simulink model "block_model"  (R2020a)
settings: Solver=VariableStepAuto  StartTime=0.0  StopTime=30  RelTol=1e-3
undefined symbols (not defined in the file or in its folder): DiscIntNeverNeededParam
libraries: simulink x6
settings Model: Creator=igorbeduin  LastModifiedBy=igorbeduin
settings SFSimCC: CustomCodeUndefinedFunction=UseInterfaceOnly

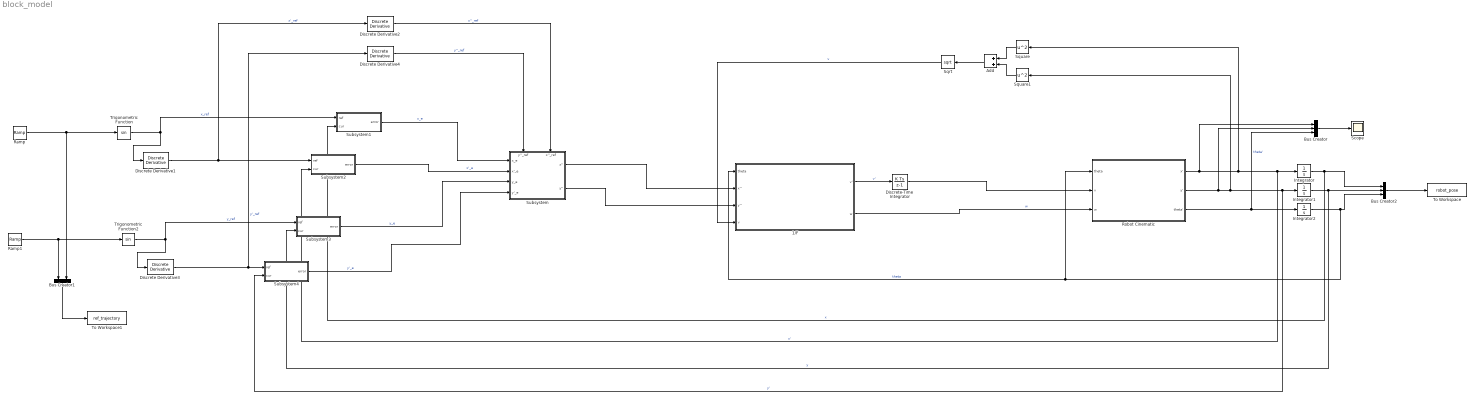
== system block_model ==
  1/F : Subsystem
  Add : Sum
  Bus Creator : BusCreator  Inputs=3
  Bus Creator1 : BusCreator  Inputs=2
  Bus Creator2 : BusCreator  Inputs=3
  Discrete Derivative{1..4} (4 alike) : simulink/Discrete/Discrete Derivative  gainval=1.0  ICPrevScaledInput=0.0  OutMin=[]  OutMax=[]  OutDataType=fixdt(1, 16)  OutScaling=2^-10  DoSatur=off
  Discrete-Time Integrator : DiscreteIntegrator  SampleTime=-1  ICPrevOutput=DiscIntNeverNeededParam  ICPrevScaledInput=DiscIntNeverNeededParam
  Integrator : Integrator
  Integrator1 : Integrator
  Integrator2 : Integrator
  Ramp : simulink/Sources/Ramp  slope=1  start=0  InitialOutput=0
  Ramp1 : simulink/Sources/Ramp  slope=2  start=0  InitialOutput=0
  Robot Cinematic : Subsystem
  Scope : Scope
  Sqrt : Sqrt  SaturateOnIntegerOverflow=on
  Square : Math  Operator=square  SaturateOnIntegerOverflow=on
  Square1 : Math  Operator=square  SaturateOnIntegerOverflow=on
  Subsystem : Subsystem
      settings: PortSchema="{\"entries\":[{\"content\":{\"sides\":[{\"content\":{\"connectorIds\":[\"In1\",\"In2\",\"In3\",\"In4\"]},\"type\":\"ConnectorPlacement.EquallySpacedRectSide\",\"uuid\":\"cf602ec4-a79b-45d8-a2b1-6ab28afdf592\"},{\"content\":{\"connectorIds\":[\"Out1\",\"Out2\"],\"side\":\"RIGHT\"},\"type\":\"ConnectorPlacement.EquallySpacedRectSide\",\"uuid\":\"65b35af8-2041-4619-9d16-3f6d6275be05\"},{\"content\":{\"connectorIds\":[\"In5\",\"In6\"],\"side\":\"TOP\"},\"type\":\"ConnectorPlacement.EquallySpacedRectSide\",\"uuid\":\"2669bffa-5f53-45fc-88ab-790e62617bda\"}]},\"type\":\"ConnectorPlacement.EquallySpacedConnector\",\"uuid\":\"c6abea3c-c3b1-4510-bea6-49383584639c\"}],\"packageUris\":[\"http://schema.mathworks.com/mf0/Connector/19700101\"],\"version\":\"1.0\"}"
  Subsystem1 : Subsystem
  Subsystem2 : Subsystem
  Subsystem3 : Subsystem
  Subsystem4 : Subsystem
  To Workspace : ToWorkspace  VariableName=robot_pose  SaveFormat=Timeseries  SampleTime=-1
  To Workspace1 : ToWorkspace  VariableName=ref_trajectory  SaveFormat=Timeseries  SampleTime=-1
  Trigonometric Function : Trigonometry
  Trigonometric Function2 : Trigonometry
  wires:
  Robot Cinematic/1(x') -> Square/1, Subsystem2/2(cur), Integrator/1, Bus Creator/1  "x'"
  Robot Cinematic/2(y') -> Square1/1, Subsystem4/2(cur), Integrator1/1, Bus Creator/2  "y'"
  Robot Cinematic/3(theta') -> Integrator2/1, Bus Creator/3  "theta'"
  1/F/1(v') -> Discrete-Time Integrator/1  "v'"
  1/F/2(w) -> Robot Cinematic/3(w)  "w"
  Integrator/1 -> Subsystem1/2(cur), Bus Creator2/1  "x"
  Integrator1/1 -> Subsystem3/2(cur), Bus Creator2/2  "y"
  Integrator2/1 -> Robot Cinematic/1(theta), 1/F/1(theta), Bus Creator2/3  "theta"
  Bus Creator/1 -> Scope/1
  Trigonometric Function/1 -> Discrete Derivative1/1, Subsystem1/1(ref)  "x_ref"
  Discrete Derivative1/1 -> Discrete Derivative2/1, Subsystem2/1(ref)  "x'_ref"
  Discrete Derivative3/1 -> Discrete Derivative4/1, Subsystem4/1(ref)  "y'_ref"
  Trigonometric Function2/1 -> Discrete Derivative3/1, Subsystem3/1(ref)  "y_ref"
  Discrete-Time Integrator/1 -> Robot Cinematic/2(v)
  Discrete Derivative2/1 -> Subsystem/6(x''_ref)  "x''_ref"
  Discrete Derivative4/1 -> Subsystem/5(y''_ref)  "y''_ref"
  Subsystem1/1(error) -> Subsystem/1(x_e)  "x_e"
  Subsystem2/1(error) -> Subsystem/2(x'_e)  "x'_e"
  Subsystem3/1(error) -> Subsystem/3(y_e)  "y_e"
  Subsystem4/1(error) -> Subsystem/4(y'_e)  "y'_e"
  Subsystem/1(x'') -> 1/F/2(x'')
  Subsystem/2(y'') -> 1/F/3(y'')
  Square/1 -> Add/1
  Square1/1 -> Add/2
  Add/1 -> Sqrt/1
  Sqrt/1 -> 1/F/4(v)  "v"
  Ramp1/1 -> Bus Creator1/1, Trigonometric Function2/1
  Ramp/1 -> Bus Creator1/2, Trigonometric Function/1
  Bus Creator2/1 -> To Workspace/1
  Bus Creator1/1 -> To Workspace1/1

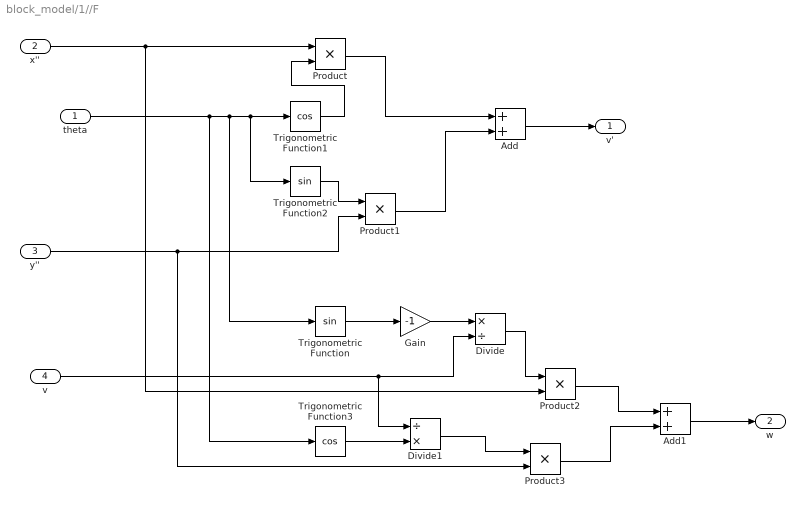
== system block_model/1//F ==
  theta : Inport
  x'' : Inport  Port=2
  y'' : Inport  Port=3
  v : Inport  Port=4
  Add : Sum
  Add1 : Sum
  Divide : Product  Inputs=*/
  Divide1 : Product  Inputs=/*
  Gain : Gain  Gain=-1
  Product{,1..3} (4 alike) : Product
  Trigonometric Function : Trigonometry
  Trigonometric Function1 : Trigonometry  Operator=cos
  Trigonometric Function2 : Trigonometry
  Trigonometric Function3 : Trigonometry  Operator=cos
  v' : Outport
  w : Outport  Port=2
  wires:
  x''/1 -> Product2/2, Product/1
  theta/1 -> Trigonometric Function/1, Trigonometric Function2/1, Trigonometric Function1/1, Trigonometric Function3/1
  Trigonometric Function1/1 -> Product/2
  Product/1 -> Add/1
  Trigonometric Function2/1 -> Product1/1
  y''/1 -> Product3/2, Product1/2
  Product1/1 -> Add/2
  Add/1 -> v'/1
  Trigonometric Function/1 -> Gain/1
  Gain/1 -> Divide/1
  v/1 -> Divide1/1, Divide/2
  Divide/1 -> Product2/1
  Product2/1 -> Add1/1
  Trigonometric Function3/1 -> Divide1/2
  Divide1/1 -> Product3/1
  Product3/1 -> Add1/2
  Add1/1 -> w/1

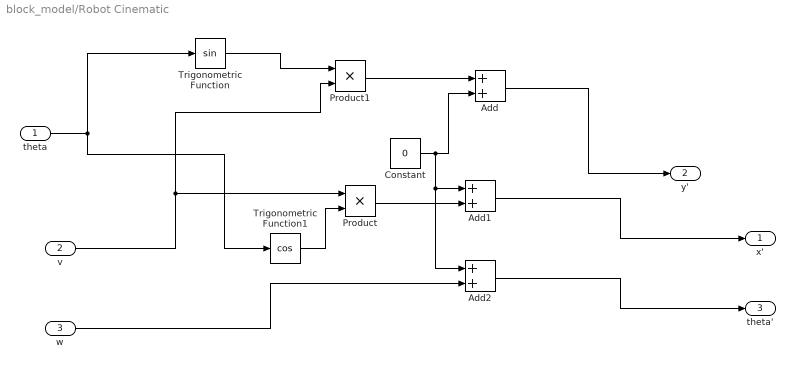
== system block_model/Robot Cinematic ==
  theta : Inport
  v : Inport  Port=2
  w : Inport  Port=3
  Add : Sum
  Add1 : Sum
  Add2 : Sum
  Constant : Constant  Value=0
  Product : Product
  Product1 : Product
  Trigonometric Function : Trigonometry
  Trigonometric Function1 : Trigonometry  Operator=cos
  x' : Outport
  y' : Outport  Port=2
  theta' : Outport  Port=3
  wires:
  theta/1 -> Trigonometric Function1/1, Trigonometric Function/1
  Trigonometric Function/1 -> Product1/1
  v/1 -> Product1/2, Product/1
  Trigonometric Function1/1 -> Product/2
  Product1/1 -> Add/1
  Constant/1 -> Add2/1, Add1/1, Add/2
  Product/1 -> Add1/2
  Add1/1 -> x'/1
  w/1 -> Add2/2
  Add2/1 -> theta'/1
  Add/1 -> y'/1

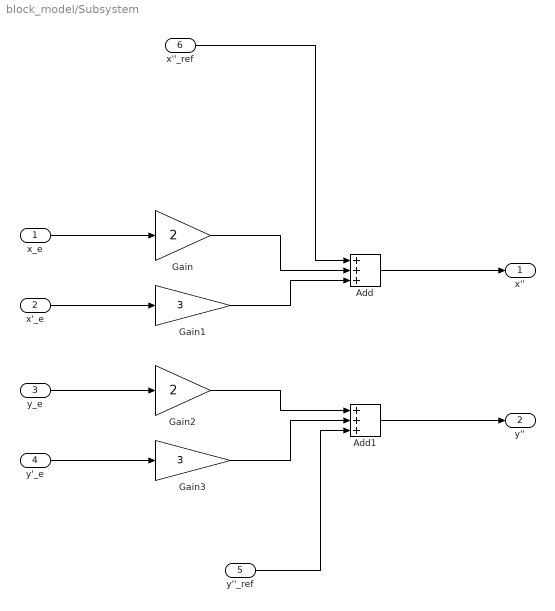
== system block_model/Subsystem ==
  x_e : Inport
  x'_e : Inport  Port=2
  y_e : Inport  Port=3
  y'_e : Inport  Port=4
  y''_ref : Inport  Port=5
  x''_ref : Inport  Port=6
  Add : Sum  Inputs=+++
  Add1 : Sum  Inputs=+++
  Gain : Gain  Gain=2
  Gain1 : Gain  Gain=3
  Gain2 : Gain  Gain=2
  Gain3 : Gain  Gain=3
  x'' : Outport
  y'' : Outport  Port=2
  wires:
  x_e/1 -> Gain/1
  x'_e/1 -> Gain1/1
  Add/1 -> x''/1
  y_e/1 -> Gain2/1
  y'_e/1 -> Gain3/1
  Add1/1 -> y''/1
  Gain1/1 -> Add/3
  Gain/1 -> Add/2
  x''_ref/1 -> Add/1
  y''_ref/1 -> Add1/3
  Gain2/1 -> Add1/1
  Gain3/1 -> Add1/2

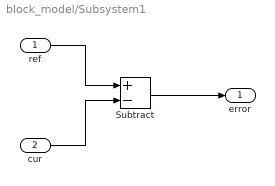
== system block_model/Subsystem1 ==
  ref : Inport
  cur : Inport  Port=2
  Subtract : Sum  Inputs=+-
  error : Outport
  wires:
  ref/1 -> Subtract/1
  cur/1 -> Subtract/2
  Subtract/1 -> error/1

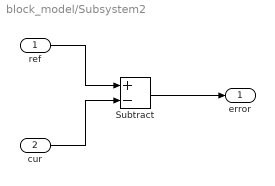
== system block_model/Subsystem2 ==
  ref : Inport
  cur : Inport  Port=2
  Subtract : Sum  Inputs=+-
  error : Outport
  wires:
  ref/1 -> Subtract/1
  cur/1 -> Subtract/2
  Subtract/1 -> error/1

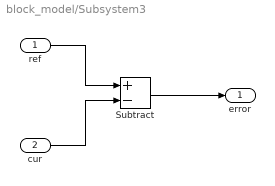
== system block_model/Subsystem3 ==
  ref : Inport
  cur : Inport  Port=2
  Subtract : Sum  Inputs=+-
  error : Outport
  wires:
  ref/1 -> Subtract/1
  cur/1 -> Subtract/2
  Subtract/1 -> error/1

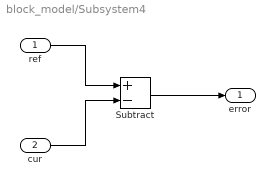
== system block_model/Subsystem4 ==
  ref : Inport
  cur : Inport  Port=2
  Subtract : Sum  Inputs=+-
  error : Outport
  wires:
  ref/1 -> Subtract/1
  cur/1 -> Subtract/2
  Subtract/1 -> error/1
